simulink model "path_detector"  (Simulink 7.6)
settings: Solver=FixedStepDiscrete  StartTime=0.0  StopTime=0  RelTol=1e-3
undefined symbols (not defined in the file or in its folder): Rec, SDTV, Track_Min_Eccentricity
libraries: vipstatistics x1, vipconversions x1, vipanalysis x1, viptransforms x1
settings Model: Creator=Thing 1  LastModifiedBy=auvt
settings OptimizationCC: OptimizeModelRefInitCode=on
settings RTWCC: SystemTargetFile=ert.tlc  GenCodeOnly=on  TemplateMakefile=ert_default_tmf  Description=Real-Time Workshop Embedded Coder  GenerateReport=on  ProcessScript=ert_make_rtw_hook  IncludeHyperlinkInReport=on  LaunchReport=on  TargetLang=C++
settings CodeAppCC: IgnoreCustomStorageClasses=off
settings ERTTargetCC: MultiwordLength=2048  GenerateSampleERTMain=on  IncludeMdlTerminateFcn=off  ERTCustomFileTemplate=example_file_process.tlc  ConvertIfToSwitch=off

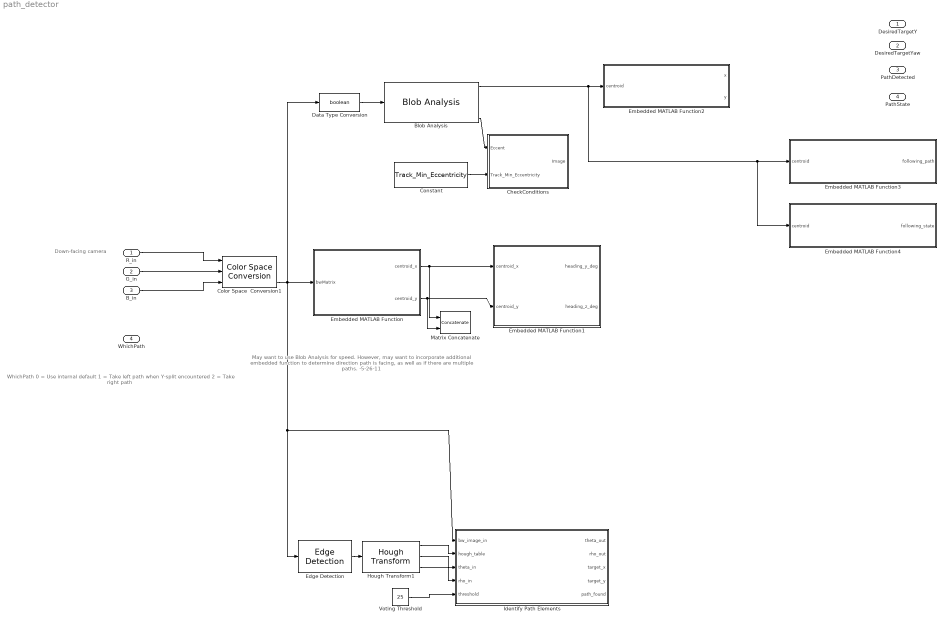
== system path_detector ==
  note: May want to use Blob Analysis for speed.
      | However, may want to incorporate
      | additional embedded function to
      | determine direction path is facing,
      | as well as if there are multiple paths.
      |
      | -5-26-11
  note: Down-facing camera
  note: WhichPath
      | 0 = Use internal default
      | 1 = Take left path when Y-split encountered
      | 2 = Take right path
  R_in : Inport  PortDimensions=Down_Camera_Dimensions
  G_in : Inport  Port=2  PortDimensions=Down_Camera_Dimensions
  B_in : Inport  Port=3  PortDimensions=Down_Camera_Dimensions
  WhichPath : Inport  Port=4
  Blob Analysis : vipstatistics/Blob Analysis  Tag=vipblks_row_conv  DialogController=vipDDGCreate  DialogControllerArgs=DataTag0  area=off  centroid=on  bBox=on  majorAxis=off  minorAxis=off  angle=on  eccentricity=on  equivDiameterSq=off  extent=off  perimeter=off  maxBlobs=Max_Num_Blobs  warnIfNumBlobsExceeded=on  isCount=off  useMinArea=on  minArea=Min_Blob_Size  useMaxArea=on  maxArea=Max_Blob_Size  excludeBorderBlob=off  outDT=double  isOutVarDim=off  isFill=on  fillValues=-1  conn=8  isLabel=off  outputMode=Binary point scaling  outputWordLength=32  outputFracLength=16  firstCoeffMode=Binary point scaling  firstCoeffWordLength=16  firstCoeffFracLength=14  secondCoeffMode=Binary point scaling  secondCoeffWordLength=32  secondCoeffFracLength=16  accumMode=Binary point scaling  accumWordLength=32  accumFracLength=0  prodOutputMode=Binary point scaling  prodOutputWordLength=32  prodOutputFracLength=16  roundingMode=Floor  overflowMode=off
  CheckConditions : Stateflow chart  TreatAsAtomicUnit=on
  Color Space  Conversion1 : vipconversions/Color Space  Conversion  conversion=Obsolete  conversionActive=R'G'B' to HSV  wp_str=D65  rec=Rec. 601 (SDTV)  sys=1125/60/2:1  imagePorts=Separate color signals
  Constant : Constant  Value=Track_Min_Eccentricity  SampleTime=-1
  Data Type Conversion : DataTypeConversion  OutDataTypeStr=boolean
  Edge Detection : vipanalysis/Edge Detection  DialogController=vipDDGCreate  DialogControllerArgs=DataTag1  method=Sobel  outputType=Binary image  userDefinedThreshold=off  thresholdSource=Specify via dialog  threshold=20  thresholdTuning=3  edgeThinning=on  threshold_canny=[0.25 0.60]  autoPercent=70  sigma=1  roundingMode=Floor  overflowMode=off
  Embedded MATLAB Function : Stateflow chart  TreatAsAtomicUnit=on
  Embedded MATLAB Function1 : Stateflow chart  TreatAsAtomicUnit=on
  Embedded MATLAB Function2 : Stateflow chart  TreatAsAtomicUnit=on
  Embedded MATLAB Function3 : Stateflow chart  TreatAsAtomicUnit=on
  Embedded MATLAB Function4 : Stateflow chart  TreatAsAtomicUnit=on
  Hough Transform1 : viptransforms/Hough Transform  DialogController=vipDDGCreate  DialogControllerArgs=DataTag2  theta_res=pi/180  rho_res=1  out_theta_rho=on  outdtmode=double  firstCoeffMode=Binary point scaling  firstCoeffWordLength=16  firstCoeffFracLength=14  secondCoeffMode=Binary point scaling  secondCoeffWordLength=32  secondCoeffFracLength=16  outputMode=Binary point scaling  outputWordLength=16  outputFracLength=0  accumMode=Binary point scaling  accumWordLength=32  accumFracLength=20  prodOutputMode=Binary point scaling  prodOutputWordLength=32  prodOutputFracLength=20  memoryMode=Binary point scaling  memoryWordLength=32  memoryFracLength=16  roundingMode=Nearest  overflowMode=on
  Identify Path Elements : Stateflow chart  TreatAsAtomicUnit=on  SystemSampleTime=[1/30 0]
  Matrix Concatenate : Concatenate  Mode=Multidimensional array  ConcatenateDimension=2
  Voting Threshold : Constant  Value=25  SampleTime=-1
  DesiredTargetY : Outport  OutDataTypeStr=double
  DesiredTargetYaw : Outport  Port=2  OutDataTypeStr=double
  PathDetected : Outport  Port=3  OutDataTypeStr=double
  PathState : Outport  Port=4  OutDataTypeStr=double
  wires:
  Constant/1 -> CheckConditions/2(Track_Min_Eccentricity)
  Embedded MATLAB Function/1(centroid_x) -> Embedded MATLAB Function1/1(centroid_x), Matrix Concatenate/1
  Embedded MATLAB Function/2(centroid_y) -> Embedded MATLAB Function1/2(centroid_y), Matrix Concatenate/2
  Blob Analysis/1 -> Embedded MATLAB Function2/1(centroid), Embedded MATLAB Function3/1(centroid), Embedded MATLAB Function4/1(centroid)
  R_in/1 -> Color Space  Conversion1/1
  B_in/1 -> Color Space  Conversion1/3
  G_in/1 -> Color Space  Conversion1/2
  Data Type Conversion/1 -> Blob Analysis/1
  Blob Analysis/4 -> CheckConditions/1(Eccent)
  Color Space  Conversion1/3 -> Embedded MATLAB Function/1(bwMatrix), Data Type Conversion/1, Edge Detection/1, Identify Path Elements/1(bw_image_in)
  Edge Detection/1 -> Hough Transform1/1
  Hough Transform1/1 -> Identify Path Elements/2(hough_table)
  Hough Transform1/2 -> Identify Path Elements/3(theta_in)
  Hough Transform1/3 -> Identify Path Elements/4(rho_in)
  Voting Threshold/1 -> Identify Path Elements/5(threshold)

== matlab function CheckConditions ==
  data: Eccent input double; Image output double; Track_Min_Eccentricity input double
function Image = CheckConditions(Eccent, Track_Min_Eccentricity)
% This function checks the conditions to decide if a track is present

if(max(abs(Eccent)) > Track_Min_Eccentricity)
    Image = 1;
else
    Image = 0;
end

return

== matlab function Embedded MATLAB Function ==
  data: bwMatrix input double; centroid_x output double; centroid_y output double

function [centroid_x, centroid_y] = CentroidVertScan(bwMatrix)

centroid_x = 0;
centroid_y = 0;

%{
%Author: Yama Habib
%Revision: 10/27/2010
%CentroidVertScan takes a black and white matrix (the expected output of
%the blob detection algorithm) with a single (rectangular) object detected,
%and returns the raw matrix coordinate of the centroid of the object. To
%convert to an angular heading, use the Centroid2Heading function.

%Should these be parameters? I think they're fine as constants.
WIDTH = size(bwMatrix, 2);
HEIGHT = size(bwMatrix, 1);

%increase the x step to increase efficiency. The further this
%number is from 1, the closer the object will have to be to be detected
%NOTE: find the max distance the hedge will be from the AUV, then find the
%optimal (lowest working) x step for that distance!
X_STEP = 1;
Y_STEP = 1;

%Don't detect lines unless they are longer than HEIGHT*THRESHOLD
THRESHOLD = 0.1;

%Allocate arrays...allocate more or less memory depending on how many lines
%are found in the average case
lineLengths = zeros(WIDTH,1);
lineMidpts_y = zeros(WIDTH,1);
lineMidpts_x = zeros(WIDTH,1);

%Find vertical lines
index = 1;
i = 1;
while(i <= WIDTH)
    j = 1;
    while(j <= HEIGHT)
        %skip whitespace
        while(bwMatrix(j,floor(i)) == 0)
%        while(bwMatrix(floor(i),j) == 0)
            j = j+1;
            if(j > HEIGHT)
                break;
            end
        end
        %count contiguous blackspace
        if(j <= HEIGHT)
            length = 0;
            midpt = j;
            while(bwMatrix(floor(i),j) ~= 0)
                length = length+1;
                j = j+1;
                if(j > HEIGHT)
                    break;
                end
            end
            midpt = midpt + length/2;
            %only register as a line if longer than HEIGHT*THRESHOLD
            if(length > HEIGHT*THRESHOLD)
                lineLengths(index) = length;
                lineMidpts_y(index) = midpt;
                lineMidpts_x(index) = floor(i);
                index = index+1;
            end
        end
        %rinse, repeat
    end
    i = i+X_STEP;
end

%Find maximum (longest rightmost) and minimum (longest leftmost) vertical
%lines
i = 1;
min = 1;
max = 1;
while(i <= index);
    
    % The following comparisons seek to minimize and maximize the metric
    %   " length*( width - x_midpt ) ". This effectively finds the largest
    %   leftmost and rightmost vertical lines.
    
    % This if statement should be "<" instead of ">" ??
    if(lineLengths(i)*(WIDTH-lineMidpts_x(i)) > lineLengths(min)*(WIDTH-lineMidpts_x(min)))
        min = i;
    end
    % This if statement should be correct
    if(lineLengths(i)*(lineMidpts_x(i)) >= lineLengths(max)*(lineMidpts_x(max)))
        max = i;
    end
    i = i+1;
end

%The centroid is (should be) the midpoint between the max's midpoint and
%the min's midpoint
% The assumption made is that the rightmost and leftmost lines bound a
% vertically-oriented rectangular path
centroid_x = (lineMidpts_x(min) + lineMidpts_x(max))/2;
centroid_y = (lineMidpts_y(min) + lineMidpts_y(max))/2;
end











%}










%{

% The following is the old code:







function [centroid_x, centroid_y] = CentroidVertScan(bwMatrix)
%Author: Yama Habib
%Revision: 10/27/2010
%CentroidVertScan takes a black and white matrix (the expected output of
%the blob detection algorithm) with a single (rectangular) object detected,
%and returns the raw matrix coordinate of the centroid of the object. To
%convert to an angular heading, use the Centroid2Heading function.

%Should these be parameters? I think they're fine as constants.
WIDTH = size(bwMatrix, 2);
HEIGHT = size(bwMatrix, 1);
%WIDTH = 160;
%HEIGHT = 120;

%increase the x step to increase efficiency. The further this
%number is from 1, the closer the object will have to be to be detected
%NOTE: find the max distance the hedge will be from the AUV, then find the
%optimal (lowest working) x step for that distance!
X_STEP = 1;

%Don't detect lines unless they are longer than HEIGHT*THRESHOLD
THRESHOLD = 0.1;

%Allocate arrays...allocate more or less memory depending on how many lines
%are found in the average case
lineLengths = zeros(WIDTH,1);
lineMidpts_y = zeros(WIDTH,1);
lineMidpts_x = zeros(WIDTH,1);

%Find vertical lines
index = 1;
i = 1;
while(i <= WIDTH)
    j = 1;
    while(j <= HEIGHT)
        %skip whitespace
        while(bwMatrix(j,floor(i)) == 0)
%        while(bwMatrix(floor(i),j) == 0)
            j = j+1;
            if(j > HEIGHT)
                break;
            end
        end
        %count contiguous blackspace
        if(j <= HEIGHT)
            length = 0;
            midpt = j;
            while(bwMatrix(floor(i),j) ~= 0)
                length = length+1;
                j = j+1;
                if(j > HEIGHT)
                    break;
                end
            end
            midpt = midpt + length/2;
            %only register as a line if longer than HEIGHT*THRESHOLD
            if(length > HEIGHT*THRESHOLD)
                lineLengths(index) = length;
                lineMidpts_y(index) = midpt;
                lineMidpts_x(index) = floor(i);
                index = index+1;
            end
        end
        %rinse, repeat
    end
    i = i+X_STEP;
end

%Find maximum (longest rightmost) and minimum (longest leftmost) vertical
%lines
i = 1;
min = 1;
max = 1;
while(i <= index);
    
    % The following comparisons seek to minimize and maximize the metric
    %   " length*( width - x_midpt ) ". This effectively finds the largest
    %   leftmost and rightmost vertical lines.
    
    % This if statement should be "<" instead of ">" ??
    if(lineLengths(i)*(WIDTH-lineMidpts_x(i)) > lineLengths(min)*(WIDTH-lineMidpts_x(min)))
        min = i;
    end
    % This if statement should be correct
    if(lineLengths(i)*(lineMidpts_x(i)) >= lineLengths(max)*(lineMidpts_x(max)))
        max = i;
    end
    i = i+1;
end

%The centroid is (should be) the midpoint between the max's midpoint and
%the min's midpoint
% The assumption made is that the rightmost and leftmost lines bound a
% vertically-oriented rectangular path
centroid_x = (lineMidpts_x(min) + lineMidpts_x(max))/2;
centroid_y = (lineMidpts_y(min) + lineMidpts_y(max))/2;
end

%}

== matlab function Embedded MATLAB Function1 ==
  data: centroid_x input double; heading_y_deg output double; centroid_y input double; heading_z_deg output double
function [heading_y_deg, heading_z_deg] = Centroid2Heading(centroid_x, centroid_y)
%Author: Yama Habib
%Revision: 10/27/2010
%Centroid2Heading takes a raw matrix centroid coordinate and converts
%it into a correction heading, in degrees (i.e. heading_y_deg = -30,
%heading_z_deg = 45 means that in order to orient yourself so that the
%object in question is centered in the video feed, you need to turn 30
%degrees to the left and 45 degrees upwards, assuming the camera is mounted
%on the front) The probability that this function will return exactly 0
%degrees is laughably low, so applying a reasonable threshold to the
%result is strongly recommended.

%Should these be parameters? I think they're fine as constants.
WIDTH = 160;
HEIGHT = 120;
MAXANGLE = 130;

heading_y_deg = ((centroid_x-(WIDTH/2)) / (WIDTH/2)) * (MAXANGLE/2);
heading_z_deg = ((centroid_y-(HEIGHT/2)) / (HEIGHT/2)) * (MAXANGLE/2);
end

== matlab function Embedded MATLAB Function2 ==
  data: x output double; centroid input double; y output double
function [x, y] = separate_centroids(centroid)

x = centroid(1);
y = centroid(2);

== matlab function Embedded MATLAB Function3 ==
  data: following_path output double; centroid input double
function following_path = separate_centroids(centroid)

% If at least one path element is found, then report that the path is being
% followed
if(size(centroid,1) ~= 0)
    following_path = 1;
else
    following_path = 0;
end

== matlab function Embedded MATLAB Function4 ==
  data: following_state output double; centroid input double
function following_state = separate_centroids(centroid)

% Editing note:
%   -centroid is not a useful input. This function has yet to be written.
%      -5-27-11


% Determine whether:
%   0 = No path is being followed
%   1 = A single path (can be made up of n path elements along one line)
%         is being followed
%   2 = A Y-split is being encountered
%   3 = A Y-join is being encountered

following_state = 1;

== matlab function Identify Path Elements ==
  data: bw_image_in input double; hough_table input double; theta_out output double; rho_out output double; target_x output double; target_y output double; path_found output double; theta_in input double; rho_in input double; threshold input double
function [theta_out, rho_out, target_x, target_y, path_found] = path_detection(bw_image_in, hough_table, theta_in, rho_in, threshold)
%#eml

% This function attempts to identfiy path elements, and returns lines,
%   targeting information, and a true/false path_found parameter.
%
% 5-30-11
%
% Input
%
% Output
%
% Notes:
%   The hough_table is destroyed in this function (acceptable if
%     hough_table is not an output)


% Initialize
peak_tol_ratio = .1;  % Fraction of max(rows,cols) of image within which a
%                         peak is assumed to reside; this helps reduce
%                         incorrect line extraction
max_num_lines = 10;  % Considers this many popular lines as candidates

[rho_length, theta_length] = size(hough_table);
[rows, cols] = size(bw_image_in);
rho_tol = .1*max(rows,cols);
theta_tol = 10*pi/180;  % Tolerence within which two slopes are equal (radians)

%rho_out = zeros(1,3);
%theta_out = zeros(1,3);
rho = zeros(1,max_num_lines);
theta = zeros(1,max_num_lines);


% Apply appropriate threshold
hough_table = hough_table.*( hough_table > threshold );


% Identify the most likely max_num_lines lines
i_index = ones(1,max_num_lines);
j_index = ones(1,max_num_lines);

m = 1;
while( m <= max_num_lines )
    
    max_votes = 0;
    for i = 1:rho_length
        for j = 1:theta_length
            if( hough_table(i,j) > max_votes )
                i_index(m) = i;
                j_index(m) = j;
                max_votes = hough_table(i,j);
            end
        end
    end
    
    rho(m) = rho_in(i_index(m));
    theta(m) = theta_in(j_index(m));
    hough_table(i_index(m),j_index(m)) = 0;
    m = m + 1;
    
end





% debug
rho_out = rho;
theta_out = theta;




% Extract the three most popular lines that fit the geometric criteria for
%   the goalpost
rho_out(1) = rho(1);
theta_out(1) = theta(1);

m = 2;
for i = 2:max_num_lines
    
    % If rho, theta do not match within tolerance, then store as the next
    %   line
    if( abs(rho(i) - rho(i-1)) >= 30 )
        rho_out(m) = rho(i);
        theta_out(m) = theta(i);
        m = m + 1;
        if( m > 3 )
            break;
        end
    end
    
end



% debug
rho_out = rho;
theta_out = theta;
target_x = 0;
target_y = 0;
path_found = 0;


return
